simulink model "Modelo_Motor"  (R2020a)
settings: Solver=VariableStepAuto  StartTime=0.0  StopTime=10  FixedStep=0.002  RelTol=1e-3
undefined symbols (not defined in the file): Ad, b_motor, bd, c, J_motor, kc, ki, Km_motor, Kt_motor, L, R_motor, T
settings Model: Creator=elkin  LastModifiedBy=elkin

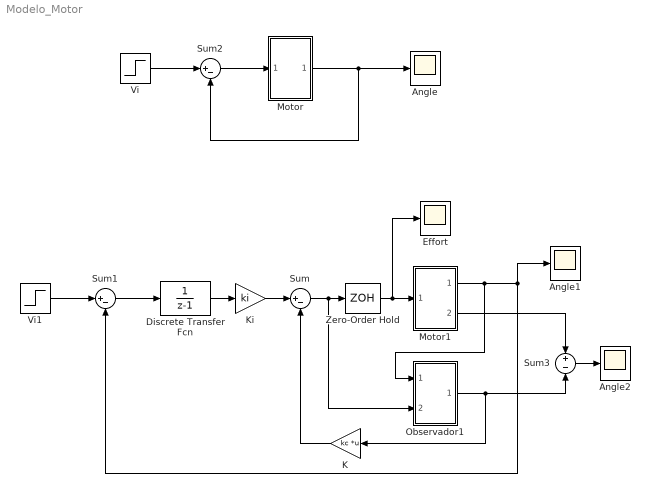
== system Modelo_Motor ==
  Angle : Scope
  Angle1 : Scope
  Angle2 : Scope
  Discrete Transfer Fcn : DiscreteTransferFcn  Denominator=[1 -1]  SampleTime=T
  Effort : Scope
  K : Gain  Gain=kc  Multiplication=Matrix(K*u)
  Ki : Gain  Gain=ki
  Motor : Subsystem
  Motor1 : Subsystem
  Observador1 : Subsystem
  Sum : Sum  Inputs=|+-
  Sum1 : Sum  Inputs=|+-
  Sum2 : Sum  Inputs=|+-
  Sum3 : Sum  Inputs=+-
  Vi : Step  Time=0  SampleTime=0
  Vi1 : Step  Time=0  SampleTime=0
  Zero-Order Hold : ZeroOrderHold  SampleTime=T
  wires:
  Vi/1 -> Sum2/1
  Motor/1(Out1) -> Sum2/2, Angle/1
  Sum2/1 -> Motor/1(In1)
  Motor1/1(Out1) -> Observador1/1(In1), Angle1/1, Sum1/2
  Zero-Order Hold/1 -> Effort/1, Motor1/1(In1)
  Sum/1 -> Observador1/2(In2), Zero-Order Hold/1
  K/1 -> Sum/2
  Vi1/1 -> Sum1/1
  Ki/1 -> Sum/1
  Sum1/1 -> Discrete Transfer Fcn/1
  Discrete Transfer Fcn/1 -> Ki/1
  Observador1/1(Out1) -> Sum3/2, K/1
  Sum3/1 -> Angle2/1
  Motor1/2(Out2) -> Sum3/1

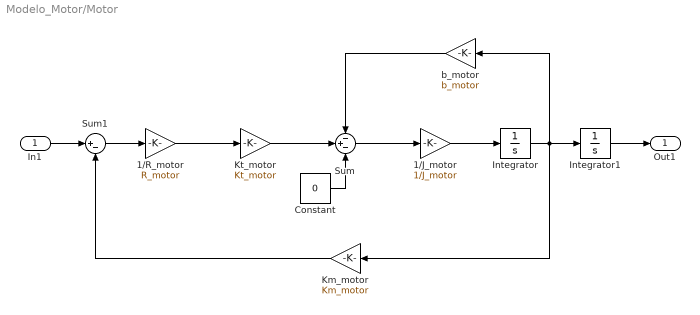
== system Modelo_Motor/Motor ==
  In1 : Inport
  1/J_motor : Gain  Gain=1/J_motor
  1/R_motor : Gain  Gain=R_motor
  Constant : Constant  Value=0
  Integrator : Integrator
  Integrator1 : Integrator
  Km_motor : Gain  Gain=Km_motor
  Kt_motor : Gain  Gain=Kt_motor
  Sum : Sum  Inputs=-+-
  Sum1 : Sum  Inputs=|+-
  b_motor : Gain  Gain=b_motor
  Out1 : Outport
  wires:
  Sum/1 -> 1/J_motor/1
  Km_motor/1 -> Sum1/2
  Constant/1 -> Sum/3
  Integrator/1 -> Km_motor/1, b_motor/1, Integrator1/1
  1/R_motor/1 -> Kt_motor/1
  Integrator1/1 -> Out1/1
  Kt_motor/1 -> Sum/2
  1/J_motor/1 -> Integrator/1
  Sum1/1 -> 1/R_motor/1
  b_motor/1 -> Sum/1
  In1/1 -> Sum1/1

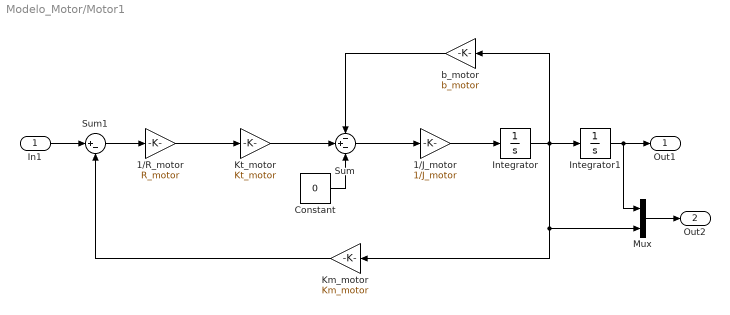
== system Modelo_Motor/Motor1 ==
  In1 : Inport
  1/J_motor : Gain  Gain=1/J_motor
  1/R_motor : Gain  Gain=R_motor
  Constant : Constant  Value=0
  Integrator : Integrator
  Integrator1 : Integrator
  Km_motor : Gain  Gain=Km_motor
  Kt_motor : Gain  Gain=Kt_motor
  Mux : Mux  Inputs=2
  Sum : Sum  Inputs=-+-
  Sum1 : Sum  Inputs=|+-
  b_motor : Gain  Gain=b_motor
  Out1 : Outport
  Out2 : Outport  Port=2
  wires:
  Sum/1 -> 1/J_motor/1
  Km_motor/1 -> Sum1/2
  Constant/1 -> Sum/3
  Integrator/1 -> Mux/2, Km_motor/1, b_motor/1, Integrator1/1
  1/R_motor/1 -> Kt_motor/1
  Integrator1/1 -> Mux/1, Out1/1
  Kt_motor/1 -> Sum/2
  1/J_motor/1 -> Integrator/1
  Sum1/1 -> 1/R_motor/1
  b_motor/1 -> Sum/1
  In1/1 -> Sum1/1
  Mux/1 -> Out2/1

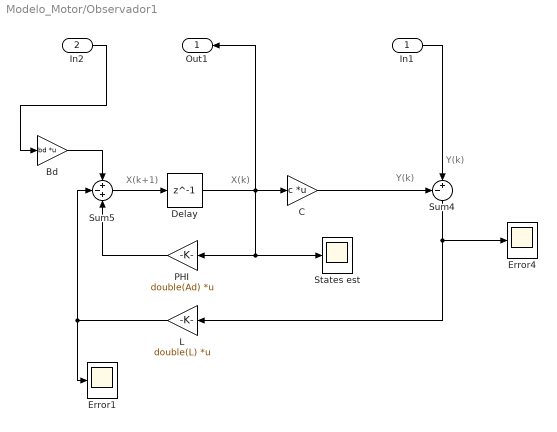
== system Modelo_Motor/Observador1 ==
  note: Y(k)
  note: X(k+1)
  note: X(k)
  note: Y(k)
  In1 : Inport
  In2 : Inport  Port=2
  Bd : Gain  Gain=bd  Multiplication=Matrix(K*u)
  C : Gain  Gain=c  Multiplication=Matrix(K*u)
  Delay : Delay  DelayLength=1  SampleTime=T
  Error1 : Scope
  Error4 : Scope
  L : Gain  Gain=double(L)  Multiplication=Matrix(K*u)
  PHI : Gain  Gain=double(Ad)  Multiplication=Matrix(K*u)
  States est : Scope
  Sum4 : Sum  Inputs=-+|
  Sum5 : Sum  Inputs=+-+
  Out1 : Outport
  wires:
  Delay/1 -> Out1/1, States est/1, PHI/1, C/1
  Sum5/1 -> Delay/1
  PHI/1 -> Sum5/3
  Sum4/1 -> Error4/1, L/1
  In2/1 -> Bd/1
  Bd/1 -> Sum5/1
  In1/1 -> Sum4/2
  L/1 -> Sum5/2, Error1/1
  C/1 -> Sum4/1
